simulink model "Euler_Test_v2"  (Simulink 7.5)
settings: Solver=FixedStepDiscrete  StartTime=0.0  StopTime=t(end)  FixedStep=SampleT  RelTol=1e-3
values from neighbouring files (symbols this model uses):
  SampleT = 0.02    [demoz2SlugsV5.m]
undefined symbols (not defined in the file or in its folder): DiscIntNeverNeededParam, ePhi_IC, Psi_IC, Theta_IC
libraries: simulink x2
settings Model: Creator=Robert  LastModifiedBy=Robert
settings DataIOCC: LimitDataPoints=off

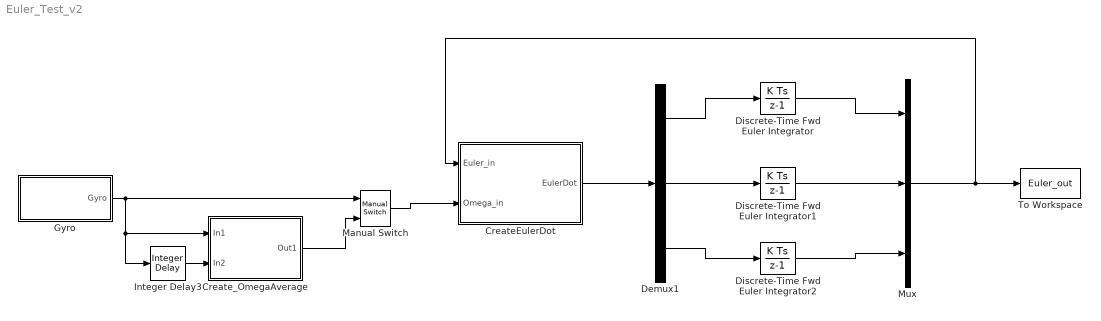
== system Euler_Test_v2 ==
  CreateEulerDot : Subsystem
  Create_OmegaAverage : Subsystem
  Demux1 : Demux  Outputs=3
  Discrete-Time Fwd Euler Integrator : DiscreteIntegrator  InitialCondition=ePhi_IC  SampleTime=SampleT  OutDataTypeMode=single  OutDataType=fixdt(1, 16)  OutScaling=2^0  OutDataTypeStr=single  ICPrevOutput=DiscIntNeverNeededParam  ICPrevScaledInput=DiscIntNeverNeededParam
  Discrete-Time Fwd Euler Integrator1 : DiscreteIntegrator  InitialCondition=Theta_IC  SampleTime=SampleT  OutDataTypeMode=single  OutDataType=fixdt(1, 16)  OutScaling=2^0  OutDataTypeStr=single  ICPrevOutput=DiscIntNeverNeededParam  ICPrevScaledInput=DiscIntNeverNeededParam
  Discrete-Time Fwd Euler Integrator2 : DiscreteIntegrator  InitialCondition=Psi_IC  SampleTime=SampleT  OutDataTypeMode=single  OutDataType=fixdt(1, 16)  OutScaling=2^0  OutDataTypeStr=single  ICPrevOutput=DiscIntNeverNeededParam  ICPrevScaledInput=DiscIntNeverNeededParam
  Gyro : Subsystem
  Integer Delay3 : simulink/Discrete/Integer Delay  vinit=0.0  samptime=-1  NumDelays=1
  Manual Switch : simulink/Signal Routing/Manual Switch  SystemSampleTime=-1  sw=0  action=0  varsize=off
  Mux : Mux  Inputs=3
  To Workspace : ToWorkspace  VariableName=Euler_out  SampleTime=SampleT  SaveFormat=Structure
  wires:
  Mux/1 -> To Workspace/1, CreateEulerDot/1(Euler_in)
  Discrete-Time Fwd Euler Integrator/1 -> Mux/1
  Discrete-Time Fwd Euler Integrator1/1 -> Mux/2
  Discrete-Time Fwd Euler Integrator2/1 -> Mux/3
  CreateEulerDot/1(EulerDot) -> Demux1/1
  Demux1/1 -> Discrete-Time Fwd Euler Integrator/1
  Demux1/2 -> Discrete-Time Fwd Euler Integrator1/1
  Demux1/3 -> Discrete-Time Fwd Euler Integrator2/1
  Manual Switch/1 -> CreateEulerDot/2(Omega_in)
  Gyro/1(Gyro) -> Manual Switch/1, Create_OmegaAverage/1(In1), Integer Delay3/1
  Integer Delay3/1 -> Create_OmegaAverage/2(In2)
  Create_OmegaAverage/1(Out1) -> Manual Switch/2

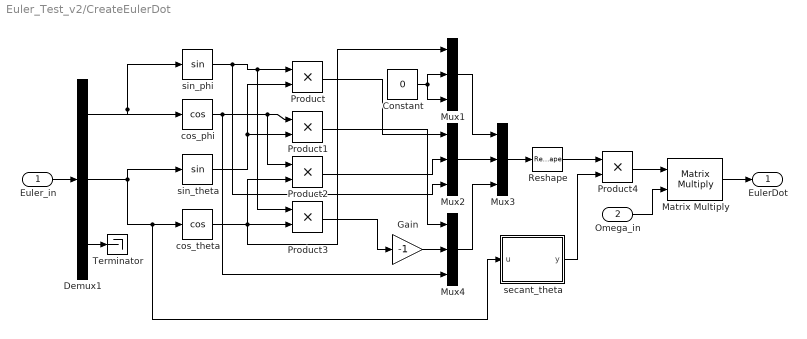
== system Euler_Test_v2/CreateEulerDot ==
  Euler_in : Inport  PortDimensions=3  SampleTime=SampleT  DataType=single  OutDataType=fixdt(1, 16)  OutScaling=2^0  OutDataTypeStr=single
  Omega_in : Inport  Port=2  PortDimensions=[3,1]  SampleTime=SampleT  DataType=single  OutDataType=fixdt(1, 16)  OutScaling=2^0  OutDataTypeStr=single
  Constant : Constant  Value=0  OutDataTypeMode=single  OutDataType=fixdt(1, 16)  OutScaling=2^0  OutDataTypeStr=single  SampleTime=SampleT
  Demux1 : Demux  Outputs=3
  Gain : Gain  Gain=-1  ParameterDataType=fixdt(1, 16)  ParameterScaling=2^0  OutDataTypeMode=single  OutDataType=fixdt(1, 16)  OutScaling=2^0  OutDataTypeStr=single  SampleTime=SampleT
  Matrix Multiply : Product  Multiplication=Matrix(*)  OutDataTypeMode=single  OutDataType=sfix(16)  OutScaling=2^0  OutDataTypeStr=single
  Mux{1..4} (4 alike) : Mux  Inputs=3
  Product{,1..3} (4 alike) : Product  OutDataTypeMode=single  OutDataType=fixdt(1, 16)  OutScaling=2^0  OutDataTypeStr=single  RndMeth=Zero
  Product4 : Product  OutDataTypeMode=single  OutDataType=fixdt(1, 16)  OutScaling=2^0  OutDataTypeStr=single  SampleTime=SampleT  RndMeth=Zero
  Reshape : Reshape  OutputDimensionality=Customize  OutputDimensions=[3,3]
  Terminator : Terminator
  cos_phi : Trigonometry  Operator=cos  SampleTime=SampleT
  cos_theta : Trigonometry  Operator=cos  SampleTime=SampleT
  secant_theta : Stateflow chart  TreatAsAtomicUnit=on
  sin_phi : Trigonometry  SampleTime=SampleT
  sin_theta : Trigonometry  SampleTime=SampleT
  EulerDot : Outport  DataType=single  OutDataType=fixdt(1, 16)  OutScaling=2^0  OutDataTypeStr=single
  wires:
  Product4/1 -> Matrix Multiply/1
  Reshape/1 -> Product4/1
  secant_theta/1(y) -> Product4/2
  Product3/1 -> Gain/1
  Gain/1 -> Mux4/2
  Product1/1 -> Mux4/1
  Product2/1 -> Mux2/2
  Product/1 -> Mux2/1
  Constant/1 -> Mux1/3, Mux1/2
  Mux4/1 -> Mux3/3
  Mux2/1 -> Mux3/2
  Mux1/1 -> Mux3/1
  Mux3/1 -> Reshape/1
  Omega_in/1 -> Matrix Multiply/2
  Matrix Multiply/1 -> EulerDot/1
  cos_theta/1 -> Mux1/1, Product3/2, Product2/2
  cos_phi/1 -> Mux4/3, Product2/1, Product1/1
  sin_theta/1 -> Product1/2, Product/2
  sin_phi/1 -> Mux2/3, Product3/1, Product/1
  Demux1/2 -> secant_theta/1(u), cos_theta/1, sin_theta/1
  Demux1/1 -> cos_phi/1, sin_phi/1
  Demux1/3 -> Terminator/1
  Euler_in/1 -> Demux1/1

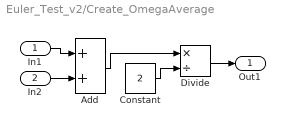
== system Euler_Test_v2/Create_OmegaAverage ==
  In1 : Inport
  In2 : Inport  Port=2
  Add : Sum  OutDataType=fixdt(1, 16)  OutScaling=2^-10
  Constant : Constant  Value=2  OutDataTypeMode=single  OutDataType=fixdt(1, 16)  OutScaling=2^0  OutDataTypeStr=single
  Divide : Product  Inputs=*/  OutDataType=fixdt(1, 16)  OutScaling=2^-10
  Out1 : Outport
  wires:
  Constant/1 -> Divide/2
  Add/1 -> Divide/1
  In1/1 -> Add/1
  In2/1 -> Add/2
  Divide/1 -> Out1/1

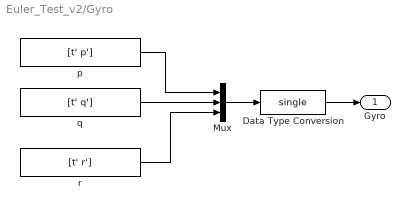
== system Euler_Test_v2/Gyro ==
  Data Type Conversion : DataTypeConversion  OutDataTypeMode=single  OutDataType=sfix(16)  OutScaling=2^0  OutDataTypeStr=single  SampleTime=SampleT
  Mux : Mux  Inputs=3
  p : FromWorkspace  VariableName=[t' p']  SampleTime=SampleT  Interpolate=off  OutputAfterFinalValue=Setting to zero
  q : FromWorkspace  VariableName=[t' q']  SampleTime=0.01  OutputAfterFinalValue=Setting to zero
  r : FromWorkspace  VariableName=[t' r']  SampleTime=0.01  OutputAfterFinalValue=Setting to zero
  Gyro : Outport  OutDataType=sfix(16)  OutScaling=2^0
  wires:
  Data Type Conversion/1 -> Gyro/1
  Mux/1 -> Data Type Conversion/1
  r/1 -> Mux/3
  q/1 -> Mux/2
  p/1 -> Mux/1

== matlab function CreateEulerDot/secant_theta ==
  data: u input double; y output double
function y = secant(u)
%#eml

y = sec(u);
